simulink model "controller_v13"  (R2020b)
settings: Solver=ode4  StartTime=0.0  StopTime=inf  RelTol=1e-3
undefined symbols (not defined in the file): ctr, DiscIntNeverNeededParam, flt, IO397, mdl, rbt, rsim, som, ukf_P0_flat, ukf_prediction_time, ukf_s0, ukf_sys, ukf_use_prediction
libraries: simulink x31, slrealtimeloglib x5, slrealtimeseriallib x5, speedgoatlib_fpga_analog_io x4, slrealtimetgmanagement x3, speedgoatlib_fpga x2, speedgoatlib_fpga_dio x1, slrealtimeutilitieslib x1
(part 1 of 5)
settings Model: SimulationMode=external  Creator=SMRL  LastModifiedBy=SMRL
settings SolverCC: ConcurrentTasks=on  PositivePriorityOrder=on  AutoInsertRateTranBlk=on
settings DataIOCC: DSMLogging=off
settings OptimizationCC: BlockReduction=off  OptimizeBlockIOStorage=off
settings DebuggingCC: TasksWithSamePriorityMsg=none
settings HardwareCC: ProdBitPerLong=64  ProdLongLongMode=on  ProdHWDeviceType=Intel->x86-64 (Linux 64)
settings RTWCC: Description=Simulink Real-Time  SystemTargetFile=slrealtime.tlc  TemplateMakefile=slrealtime_default_tmf  Toolchain=Simulink Real-Time Toolchain  BuildConfiguration=Faster Runs  CodeExecutionProfiling=on  TargetLang=C++

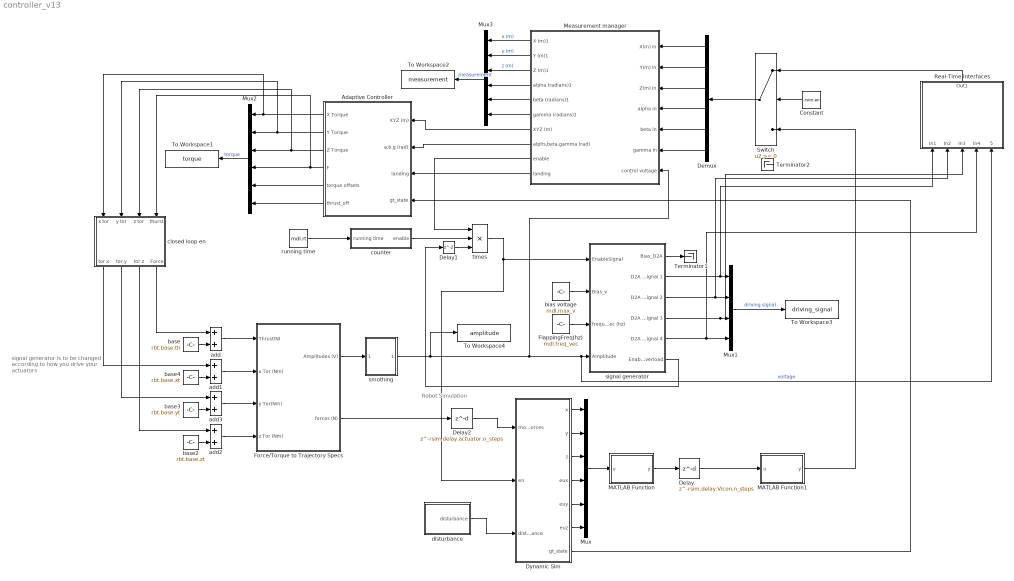
== system controller_v13 ==
  note: Robot Simulation
  note: signal generator is to be changed
      | according to how you drive your
      | actuators
  Adaptive Controller : Subsystem
  Constant : Constant  Value=-rsim.en
  Delay : Delay  DelayLength=rsim.delay.Vicon.n_steps  InitialCondition=rsim.delay.Vicon.init_val
  Delay1 : Delay  InitialCondition=1
  Delay2 : Delay  DelayLength=rsim.delay.actuator.n_steps  InitialCondition=rsim.delay.actuator.init_val
  Demux : Demux  Outputs=6
  Dynamic Sim : Subsystem  TreatAsAtomicUnit=on  SystemSampleTime=rsim.mdl.T
  FlappingFreq(hz) : Constant  Value=mdl.freq_vec  SampleTime=-1
  Force/Torque to Trajectory Specs : Subsystem
  MATLAB Function : MATLAB Function  TreatAsAtomicUnit=on  SystemSampleTime=0.001
  MATLAB Function1 : MATLAB Function  TreatAsAtomicUnit=on  SystemSampleTime=1/1000
  Measurement manager : Subsystem
  Mux : Mux  Inputs=6
  Mux1 : Mux
  Mux2 : Mux  Inputs=6
  Mux3 : Mux  Inputs=6
  Real-Time Interfaces : Subsystem
  Switch : Switch
  Terminator1 : Terminator
  Terminator2 : Terminator
  To Workspace1 : ToWorkspace  VariableName=torque  SaveFormat=Timeseries  SampleTime=-1
  To Workspace2 : ToWorkspace  VariableName=measurement  SaveFormat=Timeseries  SampleTime=-1
  To Workspace3 : ToWorkspace  VariableName=driving_signal  SaveFormat=Timeseries  SampleTime=-1
  To Workspace4 : ToWorkspace  VariableName=amplitude  SaveFormat=Timeseries  SampleTime=-1
  add{,1..3} (4 alike) : Sum
  base : Constant  Value=rbt.base.th
  base2 : Constant  Value=rbt.base.zt
  base3 : Constant  Value=rbt.base.yt
  base4 : Constant  Value=rbt.base.xt
  bias voltage : Constant  Value=mdl.max_v
  closed loop en : Subsystem
  counter : Subsystem
  disturbance : Subsystem  TreatAsAtomicUnit=on  SystemSampleTime=rsim.mdl.T
  running time : Constant  Value=mdl.rt  SampleTime=-1
  signal generator : Subsystem  TreatAsAtomicUnit=on  SystemSampleTime=mdl.T_high
  smothing : Subsystem
  times : Product  Inputs=3  RndMeth=Zero
  wires:
  add3/1 -> Force/Torque to Trajectory Specs/3(y Tor(Nm))
  Force/Torque to Trajectory Specs/2(forces (N)) -> Delay2/1
  Adaptive Controller/3(Z Torque) -> closed loop en/3(z tor), Mux2/3
  Mux3/1 -> To Workspace2/1  "measurement"
  Adaptive Controller/2(Y Torque) -> closed loop en/2(y tor), Mux2/2
  Adaptive Controller/1(X Torque) -> closed loop en/1(x tor), Mux2/1
  signal generator/5(D2A DriveSignal 4) -> Mux1/4, Real-Time Interfaces/4(In4)
  Adaptive Controller/5(" torque offsets") -> Mux2/5
  Measurement manager/5(beta (radians)1) -> Mux3/5
  signal generator/4(D2A DriveSignal 3) -> Real-Time Interfaces/3(In3), Mux1/3
  Adaptive Controller/4(" F") -> closed loop en/4(thurst), Mux2/4
  Measurement manager/6(gamma (radians)1) -> Mux3/6
  add2/1 -> Force/Torque to Trajectory Specs/4(z Tor (Nm))
  Measurement manager/4(alpha (radians)1) -> Mux3/4
  Adaptive Controller/6(thrust_off) -> Mux2/6
  closed loop en/1(tor x) -> add1/1
  base3/1 -> add3/2
  base2/1 -> add2/2
  Mux1/1 -> To Workspace3/1  "driving signal"
  closed loop en/4(Force) -> add/1
  base/1 -> add/2
  Measurement manager/8(alphs,beta,gamma (rad)) -> Adaptive Controller/2(a,b,g (rad))
  signal generator/2(D2A DriveSignal 1) -> Real-Time Interfaces/1(In1), Mux1/1
  closed loop en/2(tor y) -> add3/1
  signal generator/3(D2A DriveSignal 2) -> Mux1/2, Real-Time Interfaces/2(In2)
  Force/Torque to Trajectory Specs/1(Amplitudes (V)) -> smothing/1(amp)
  FlappingFreq(hz)/1 -> signal generator/3(frequency_vec (hz))
  Measurement manager/1(X (m)1) -> Mux3/1  "x (m)"
  Measurement manager/7(XYZ (m)) -> Adaptive Controller/1(XYZ (m))
  Measurement manager/3(Z (m)1) -> Mux3/3  "z (m)"
  base4/1 -> add1/2
  closed loop en/3(tor z) -> add2/1
  add1/1 -> Force/Torque to Trajectory Specs/2(x Tor (Nm))
  bias voltage/1 -> signal generator/2(Bias_v)
  counter/1(enable) -> times/2
  add/1 -> Force/Torque to Trajectory Specs/1(Thrust(N))
  Measurement manager/2(Y (m)1) -> Mux3/2  "y (m)"
  running time/1 -> counter/1(running time)
  Mux2/1 -> To Workspace1/1  "torque"
  signal generator/1(Bias_D2A) -> Terminator1/1
  Dynamic Sim/3(z) -> Mux/3
  Dynamic Sim/2(y) -> Mux/2
  Dynamic Sim/1(x) -> Mux/1
  Dynamic Sim/4(eux) -> Mux/4
  Dynamic Sim/5(euy) -> Mux/5
  Dynamic Sim/6(euz) -> Mux/6
  Demux/1 -> Measurement manager/1(X(m) in)
  Demux/2 -> Measurement manager/2(Y(m) in)
  Demux/3 -> Measurement manager/3(Z(m) in)
  Demux/4 -> Measurement manager/4(alpha in)
  Demux/5 -> Measurement manager/5(beta in)
  Demux/6 -> Measurement manager/6(gamma in)
  Constant/1 -> Switch/2
  disturbance/1(disturbance) -> Dynamic Sim/3(disturbance)
  Switch/1 -> Demux/1
  Delay/1 -> MATLAB Function1/1(u)
  Measurement manager/10(landing) -> Adaptive Controller/3(landing)
  signal generator/6(Enable overload) -> Delay1/1
  Delay1/1 -> times/3
  smothing/1(control voltage) -> Real-Time Interfaces/5(voltage), signal generator/4(Amplitude), Measurement manager/7(control voltage), To Workspace4/1  "voltage"
  Measurement manager/9(enable) -> times/1
  Mux/1 -> MATLAB Function/1(u)
  MATLAB Function/1(y) -> Delay/1
  MATLAB Function1/1(y) -> Switch/3
  Delay2/1 -> Dynamic Sim/1(module forces)
  Dynamic Sim/7(gt_state) -> Adaptive Controller/4(gt_state)
  times/1 -> Dynamic Sim/2(en), signal generator/1(EnableSignal)
  Real-Time Interfaces/1(Out1) -> Switch/1

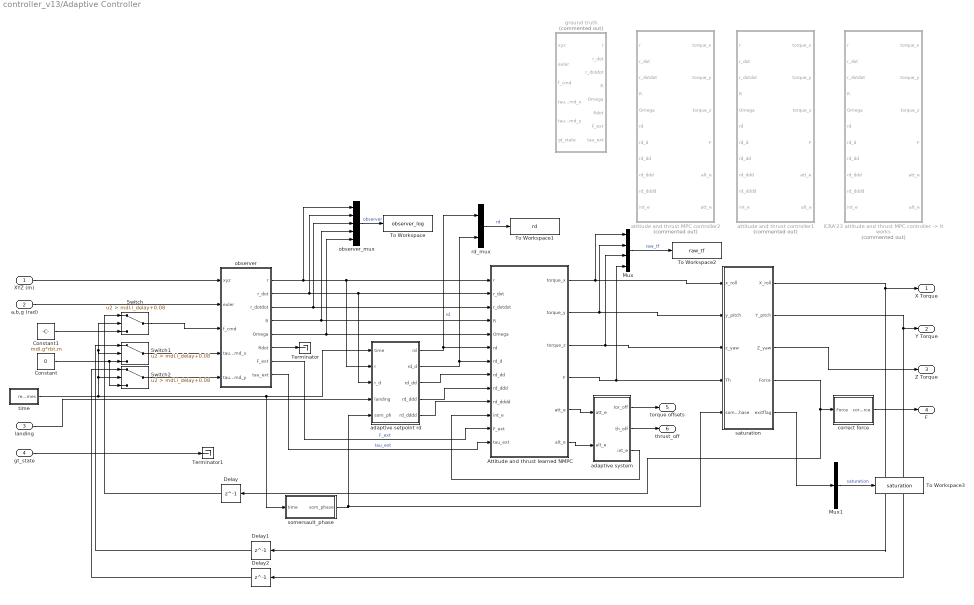
== system controller_v13/Adaptive Controller ==
  XYZ (m) : Inport
  a,b,g (rad) : Inport  Port=2
  landing : Inport  Port=3
  gt_state : Inport  Port=4
  Attitude and thrust learned NMPC : Subsystem
  Constant : Constant  Value=0
  Constant1 : Constant  Value=mdl.g*rbt.m
  Delay : Delay  DelayLength=1
  Delay1 : Delay  DelayLength=1
  Delay2 : Delay  DelayLength=1
  "ICRA'23 attitude and thrust MPC controller -> It works" : Subsystem  Commented=on
  Mux : Mux
  Mux1 : Mux  Inputs=1
  Switch : Switch  Criteria=u2 > Threshold  Threshold=mdl.i_delay+0.08
  Switch1 : Switch  Criteria=u2 > Threshold  Threshold=mdl.i_delay+0.08
  Switch2 : Switch  Criteria=u2 > Threshold  Threshold=mdl.i_delay+0.08
  Terminator : Terminator
  Terminator1 : Terminator
  To Workspace : ToWorkspace  VariableName=observer_log  SaveFormat=Timeseries  SampleTime=-1
  To Workspace1 : ToWorkspace  VariableName=rd  SaveFormat=Timeseries  SampleTime=-1
  To Workspace2 : ToWorkspace  VariableName=raw_tf  SaveFormat=Timeseries  SampleTime=-1
  To Workspace3 : ToWorkspace  VariableName=saturation  SaveFormat=Timeseries  SampleTime=-1
  adaptive setpoint rd : MATLAB Function  TreatAsAtomicUnit=on  SystemSampleTime=mdl.T
  adaptive system : Subsystem
  attitude and thrust MPC controller2 : Subsystem  Commented=on
  attitude and thrust controller1 : Subsystem  Commented=on
  correct force : MATLAB Function  TreatAsAtomicUnit=on
  ground truth : Subsystem  Commented=on
  observer : Subsystem
  observer_mux : Mux  Inputs=5
  rd_mux : Mux  Inputs=2
  saturation : MATLAB Function  TreatAsAtomicUnit=on  SystemSampleTime=mdl.T
  somersault_phase : MATLAB Function  TreatAsAtomicUnit=on
  time : Subsystem
  X Torque : Outport
  Y Torque : Outport  Port=2
  Z Torque : Outport  Port=3
  " F" : Outport  Port=4
  " torque offsets" : Outport  Port=5
  thrust_off : Outport  Port=6
  wires:
  XYZ (m)/1 -> observer/1(xyz)
  observer/2(r_dot) -> Attitude and thrust learned NMPC/2(r_dot), adaptive setpoint rd/3(r_d), observer_mux/2
  observer/3(r_dotdot) -> Attitude and thrust learned NMPC/3(r_dotdot), observer_mux/3
  a,b,g (rad)/1 -> observer/2(euler)
  observer/4(R) -> Attitude and thrust learned NMPC/4(R), observer_mux/4
  saturation/1(X_roll) -> Delay1/1, X Torque/1
  saturation/2(Y_pitch) -> Delay2/1, Y Torque/1
  saturation/3(Z_yaw) -> Z Torque/1
  saturation/4(Force) -> Delay/1, correct force/1(Force)
  Attitude and thrust learned NMPC/4(F) -> Mux/4, saturation/4(Th)
  Attitude and thrust learned NMPC/5(att_e) -> adaptive system/1(att_e)
  adaptive system/1(" tor_off") -> " torque offsets"/1
  adaptive system/2(th_off) -> thrust_off/1
  adaptive system/3(int_e) -> Attitude and thrust learned NMPC/11(int_e)
  adaptive setpoint rd/1(rd) -> Attitude and thrust learned NMPC/6(rd), rd_mux/1  "rd"
  adaptive setpoint rd/2(rd_d) -> Attitude and thrust learned NMPC/7(rd_d), rd_mux/2
  adaptive setpoint rd/3(rd_dd) -> Attitude and thrust learned NMPC/8(rd_dd)
  adaptive setpoint rd/4(rd_ddd) -> Attitude and thrust learned NMPC/9(rd_ddd)
  adaptive setpoint rd/5(rd_dddd) -> Attitude and thrust learned NMPC/10(rd_dddd)
  time/1(real times) -> Switch2/2, Switch/2, Switch1/2, somersault_phase/1(time), adaptive setpoint rd/1(time)
  Attitude and thrust learned NMPC/3(torque_z) -> Mux/3, saturation/3(z_yaw)
  Attitude and thrust learned NMPC/2(torque_y) -> Mux/2, saturation/2(y_pitch)
  Attitude and thrust learned NMPC/1(torque_x) -> Mux/1, saturation/1(x_roll)
  observer/6(Rdot) -> Terminator/1
  observer/5(Omega) -> Attitude and thrust learned NMPC/5(Omega), observer_mux/5
  Attitude and thrust learned NMPC/6(alt_e) -> adaptive system/2(alt_e)
  somersault_phase/1(som_phase) -> saturation/5(som_phase), adaptive setpoint rd/5(som_ph)
  landing/1 -> adaptive setpoint rd/4(landing)
  observer_mux/1 -> To Workspace/1  "observer"
  rd_mux/1 -> To Workspace1/1  "rd"
  Delay/1 -> Switch/1
  observer/1(r) -> Attitude and thrust learned NMPC/1(r), adaptive setpoint rd/2(r), observer_mux/1
  Delay1/1 -> Switch1/1
  Delay2/1 -> Switch2/1
  Constant/1 -> Switch2/3, Switch1/3
  Switch1/1 -> observer/4(tau_cmd_x)
  Switch/1 -> observer/3(f_cmd)
  Constant1/1 -> Switch/3
  observer/7(F_ext) -> Attitude and thrust learned NMPC/12(F_ext)  "F_ext"
  observer/8(tau_ext) -> Attitude and thrust learned NMPC/13(tau_ext)  "tau_ext"
  gt_state/1 -> Terminator1/1
  Switch2/1 -> observer/5(tau_cmd_y)
  Mux/1 -> To Workspace2/1  "raw_tf"
  saturation/5(exitflag) -> Mux1/1
  Mux1/1 -> To Workspace3/1  "saturation"
  correct force/1(corrected_force) -> " F"/1

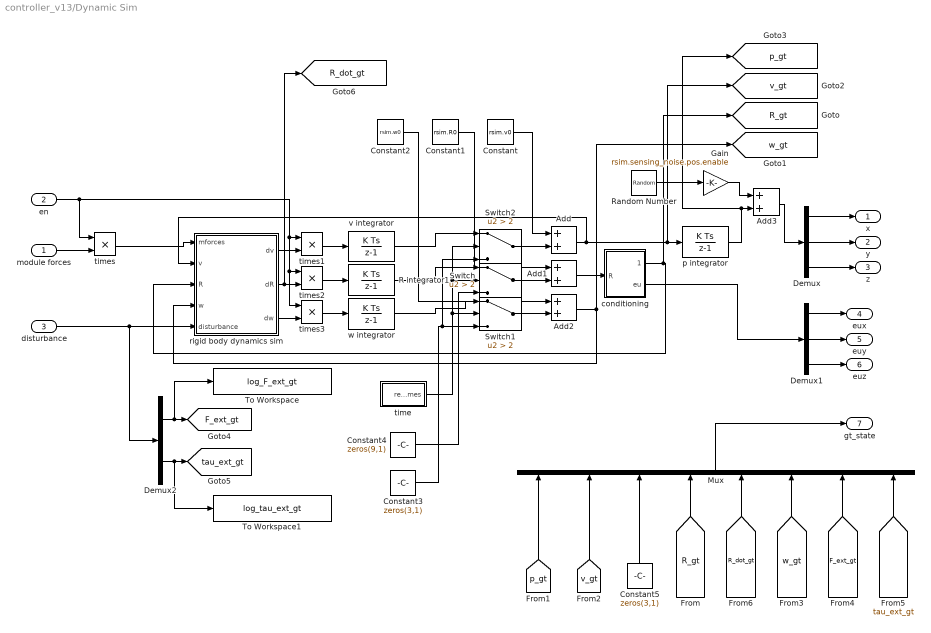
== system controller_v13/Dynamic Sim ==
  module forces : Inport
  en : Inport  Port=2
  disturbance : Inport  Port=3
  Add{,1..3} (4 alike) : Sum
  Constant : Constant  Value=rsim.v0
  Constant1 : Constant  Value=rsim.R0
  Constant2 : Constant  Value=rsim.w0
  Constant3 : Constant  Value=zeros(3,1)
  Constant4 : Constant  Value=zeros(9,1)
  Constant5 : Constant  Value=zeros(3,1)
  Demux : Demux  Outputs=3
  Demux1 : Demux  Outputs=3
  Demux2 : Demux  Outputs=[3, 3]
  Gain : Gain  Gain=rsim.sensing_noise.pos.enable
  Mux : Mux  Inputs=8
  R integrator1 : DiscreteIntegrator  gainval=1  SampleTime=-1  UpperSaturationLimit=1  LowerSaturationLimit=0  ICPrevOutput=DiscIntNeverNeededParam  ICPrevScaledInput=DiscIntNeverNeededParam
  Random Number : RandomNumber  Mean=zeros(3,1)  Variance=rsim.sensing_noise.pos_sigma.^2  SampleTime=rsim.mdl.T
  Switch : Switch  Criteria=u2 > Threshold  Threshold=2
  Switch1 : Switch  Criteria=u2 > Threshold  Threshold=2
  Switch2 : Switch  Criteria=u2 > Threshold  Threshold=2
  To Workspace : ToWorkspace  VariableName=log_F_ext_gt  SaveFormat=Timeseries  SampleTime=-1
  To Workspace1 : ToWorkspace  VariableName=log_tau_ext_gt  SaveFormat=Timeseries  SampleTime=-1
  conditioning : MATLAB Function  TreatAsAtomicUnit=on
  p integrator : DiscreteIntegrator  gainval=1  InitialCondition=rsim.p0  SampleTime=-1  UpperSaturationLimit=1  LowerSaturationLimit=0  ICPrevOutput=DiscIntNeverNeededParam  ICPrevScaledInput=DiscIntNeverNeededParam
  rigid body dynamics sim : MATLAB Function  TreatAsAtomicUnit=on
  time : Subsystem
  times{,1..3} (4 alike) : Product  RndMeth=Zero
  v integrator : DiscreteIntegrator  gainval=1  SampleTime=-1  UpperSaturationLimit=1  LowerSaturationLimit=0  ICPrevOutput=DiscIntNeverNeededParam  ICPrevScaledInput=DiscIntNeverNeededParam
  w integrator : DiscreteIntegrator  gainval=1  SampleTime=-1  UpperSaturationLimit=1  LowerSaturationLimit=0  ICPrevOutput=DiscIntNeverNeededParam  ICPrevScaledInput=DiscIntNeverNeededParam
  x : Outport  VectorParamsAs1DForOutWhenUnconnected=off
  y : Outport  Port=2  VectorParamsAs1DForOutWhenUnconnected=off
  z : Outport  Port=3  VectorParamsAs1DForOutWhenUnconnected=off
  eux : Outport  Port=4  VectorParamsAs1DForOutWhenUnconnected=off
  euy : Outport  Port=5  VectorParamsAs1DForOutWhenUnconnected=off
  euz : Outport  Port=6  VectorParamsAs1DForOutWhenUnconnected=off
  gt_state : Outport  Port=7
  tag scope: F_ext_gt=global, R_dot_gt=global, R_gt=global, p_gt=global, tau_ext_gt=global, v_gt=global, w_gt=global
  wires:
  Demux1/1 -> eux/1
  Demux1/2 -> euy/1
  Demux/3 -> z/1
  conditioning/2(eu) -> Demux1/1
  conditioning/1(R_norm_flat) -> [R_gt], rigid body dynamics sim/3(R)
  p integrator/1 -> [p_gt], Add3/2
  Demux1/3 -> euz/1
  Demux/1 -> x/1
  Demux/2 -> y/1
  Constant/1 -> Add/1
  Constant1/1 -> Add1/1
  Constant2/1 -> Add2/1
  Add1/1 -> conditioning/1(R)
  Add2/1 -> [w_gt], rigid body dynamics sim/4(w)
  Add/1 -> rigid body dynamics sim/2(v), [v_gt], p integrator/1
  en/1 -> times2/1, times3/1, times1/1, times/1
  module forces/1 -> times/2
  times/1 -> rigid body dynamics sim/1(mforces)
  times1/1 -> v integrator/1
  rigid body dynamics sim/1(dv) -> times1/2
  rigid body dynamics sim/2(dR) -> [R_dot_gt], times2/2
  rigid body dynamics sim/3(dw) -> times3/2
  times2/1 -> R integrator1/1
  times3/1 -> w integrator/1
  disturbance/1 -> Demux2/1, rigid body dynamics sim/5(disturbance)
  Random Number/1 -> Gain/1
  Gain/1 -> Add3/1
  Add3/1 -> Demux/1
  Switch2/1 -> Add/2
  Switch/1 -> Add1/2
  Switch1/1 -> Add2/2
  time/1(real times) -> Switch1/2, Switch2/2, Switch/2
  v integrator/1 -> Switch2/1
  R integrator1/1 -> Switch/1
  w integrator/1 -> Switch1/1
  Constant4/1 -> Switch/3
  Constant3/1 -> Switch2/3, Switch1/3
  Demux2/1 -> To Workspace/1, [F_ext_gt]
  Demux2/2 -> To Workspace1/1, [tau_ext_gt]
  [p_gt] -> Mux/1
  [v_gt] -> Mux/2
  Constant5/1 -> Mux/3
  [R_gt] -> Mux/4
  [R_dot_gt] -> Mux/5
  [w_gt] -> Mux/6
  [F_ext_gt] -> Mux/7
  [tau_ext_gt] -> Mux/8
  Mux/1 -> gt_state/1

== system controller_v13/Force//Torque to Trajectory Specs ==
  Thrust(N) : Inport
  x Tor (Nm) : Inport  Port=2
  y Tor(Nm) : Inport  Port=3
  z Tor (Nm) : Inport  Port=4
  force/torque to module thrust : Subsystem
  nominal desired voltage : Subsystem
  Amplitudes (V) : Outport
  forces (N) : Outport  Port=2
  wires:
  Thrust(N)/1 -> force/torque to module thrust/1(thrust)
  y Tor(Nm)/1 -> force/torque to module thrust/3(y Tq)
  z Tor (Nm)/1 -> force/torque to module thrust/4(z Tq)
  force/torque to module thrust/1(module thrusts (1-4)) -> forces (N)/1, nominal desired voltage/1(Force)
  x Tor (Nm)/1 -> force/torque to module thrust/2(x Tq)
  nominal desired voltage/1(Voltages) -> Amplitudes (V)/1

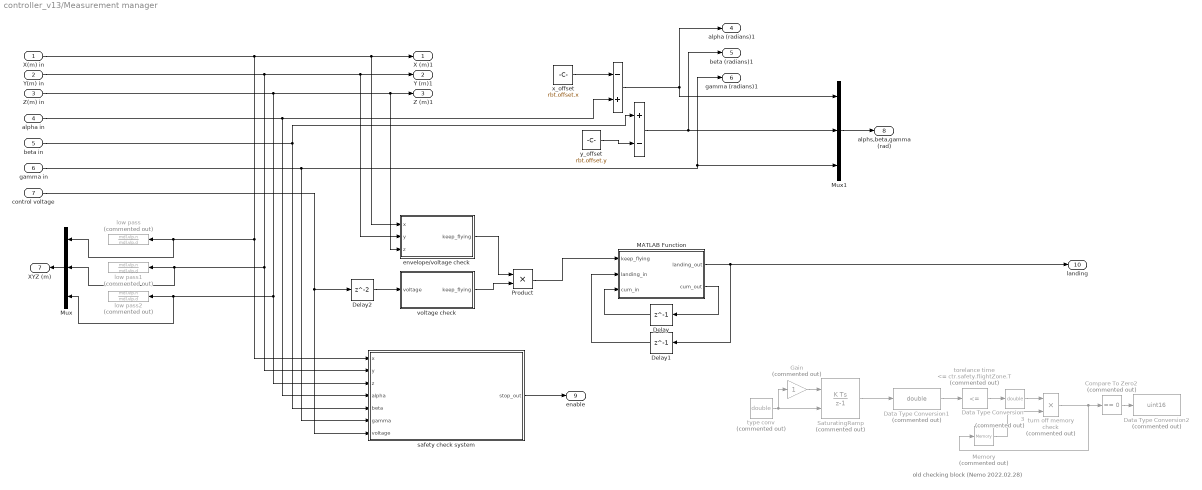
== system controller_v13/Measurement manager ==
  note: old checking block (Nemo 2022.02.28)
  X(m) in : Inport
  Y(m) in : Inport  Port=2
  Z(m) in : Inport  Port=3
  alpha in : Inport  Port=4
  beta in : Inport  Port=5
  gamma in : Inport  Port=6
  control voltage : Inport  Port=7
  " " : Sum  Inputs=-+
  "  " : Sum  Inputs=+-
  Compare To Zero2 : simulink/Logic and Bit Operations/Compare To Zero  Commented=on  relop===  OutDataTypeStr=uint8
  Data Type Conversion1 : DataTypeConversion  Commented=on  OutDataTypeStr=double
  Data Type Conversion2 : DataTypeConversion  Commented=on  OutDataTypeStr=uint16
  Data Type Conversion3 : DataTypeConversion  Commented=on  OutDataTypeStr=double
  Delay : Delay  DelayLength=1
  Delay1 : Delay  DelayLength=1
  Delay2 : Delay
  Gain : Gain  Commented=on
  MATLAB Function : MATLAB Function  TreatAsAtomicUnit=on
  Memory : Memory  Commented=on  InitialCondition=1
  Mux : Mux  Inputs=3
  Mux1 : Mux  Inputs=3
  Product : Product
  SaturatingRamp : DiscreteIntegrator  Commented=on  gainval=1  ExternalReset=falling  SampleTime=-1  UpperSaturationLimit=1  LowerSaturationLimit=0  ICPrevOutput=DiscIntNeverNeededParam  ICPrevScaledInput=DiscIntNeverNeededParam
  envelope/voltage check : MATLAB Function  TreatAsAtomicUnit=on
  low pass : DiscreteTransferFcn  Commented=on  Numerator=mdl.vlp.n  Denominator=mdl.vlp.d
  low pass1 : DiscreteTransferFcn  Commented=on  Numerator=mdl.vlp.n  Denominator=mdl.vlp.d
  low pass2 : DiscreteTransferFcn  Commented=on  Numerator=mdl.vlp.n  Denominator=mdl.vlp.d
  safety check system : Subsystem
  torelance time : simulink/Logic and Bit Operations/Compare To Constant  Commented=on  relop=<=  const=ctr.safety.flightZone.T  OutDataTypeStr=uint8
  turn off memory check : Product  Commented=on  RndMeth=Zero
  type conv : DataTypeConversion  Commented=on  OutDataTypeStr=double
  voltage check : MATLAB Function  TreatAsAtomicUnit=on  SystemSampleTime=mdl.T
  x_offset : Constant  Value=rbt.offset.x
  y_offset : Constant  Value=rbt.offset.y
  X (m)1 : Outport
  Y (m)1 : Outport  Port=2
  Z (m)1 : Outport  Port=3
  alpha (radians)1 : Outport  Port=4
  beta (radians)1 : Outport  Port=5
  gamma (radians)1 : Outport  Port=6
  XYZ (m) : Outport  Port=7
  alphs,beta,gamma (rad) : Outport  Port=8
  enable : Outport  Port=9
  landing : Outport  Port=10
  wires:
  X(m) in/1 -> safety check system/1(x), Mux/1, low pass/1, envelope/voltage check/1(x), X (m)1/1
  Y(m) in/1 -> safety check system/2(y), Mux/2, low pass1/1, envelope/voltage check/2(y), Y (m)1/1
  Z(m) in/1 -> safety check system/3(z), Mux/3, low pass2/1, envelope/voltage check/3(z), Z (m)1/1
  alpha in/1 -> safety check system/4(alpha), " "/2
  beta in/1 -> "  "/1, safety check system/5(beta)
  Mux/1 -> XYZ (m)/1
  Mux1/1 -> alphs,beta,gamma (rad)/1
  y_offset/1 -> "  "/2
  x_offset/1 -> " "/1
  control voltage/1 -> Delay2/1, safety check system/7(voltage)
  safety check system/1(stop_out) -> enable/1
  Gain/1 -> SaturatingRamp/1
  Data Type Conversion3/1 -> turn off memory check/1
  Data Type Conversion1/1 -> torelance time/1
  type conv/1 -> SaturatingRamp/2, Gain/1
  SaturatingRamp/1 -> Data Type Conversion1/1
  torelance time/1 -> Data Type Conversion3/1
  turn off memory check/1 -> Compare To Zero2/1, Memory/1
  Memory/1 -> turn off memory check/2
  Compare To Zero2/1 -> Data Type Conversion2/1
  " "/1 -> Mux1/1, alpha (radians)1/1
  "  "/1 -> beta (radians)1/1, Mux1/2
  gamma in/1 -> Mux1/3, gamma (radians)1/1, safety check system/6(gamma)
  Delay/1 -> MATLAB Function/3(cum_in)
  MATLAB Function/2(cum_out) -> Delay/1
  MATLAB Function/1(landing_out) -> Delay1/1, landing/1
  Delay1/1 -> MATLAB Function/2(landing_in)
  envelope/voltage check/1(keep_flying) -> Product/1
  Delay2/1 -> voltage check/1(voltage)
  voltage check/1(keep_flying) -> Product/2
  Product/1 -> MATLAB Function/1(keep_flying)

== system controller_v13/Real-Time Interfaces ==
  In1 : Inport
  In2 : Inport  Port=2
  In3 : Inport  Port=3
  In4 : Inport  Port=4
  voltage : Inport  Port=5
  Cast To Double : DataTypeConversion  OutDataTypeStr=double
  Constant1 : Constant  Value=mdl.i_delay
  Digital output : speedgoatlib_fpga_dio/Digital output  id=2  chan=[7]  init=[0]  reset=[0]  vectorizeInput=off  ts=mdl.T  pciSlot=[11,0]  board=IO397-50k
      settings: SourceProductName=Simulink Real-Time: Speedgoat I/O Driver Library
  IO397 Analog Output : speedgoatlib_fpga_analog_io/IO397 Analog Output  id=1  chan=1:2  initVal=0  resetVal=0  ts=-1  pciSlot=[6,0]  board=IO397-50k  span=+10.8 V
      settings: SourceProductName=Simulink Real-Time: Speedgoat Library
  IO397 Analog Output1 : speedgoatlib_fpga_analog_io/IO397 Analog Output  id=2  chan=1:2  initVal=0  resetVal=0  ts=-1  pciSlot=[11,0]  board=IO397-50k  span=+10.8 V
      settings: SourceProductName=Simulink Real-Time: Speedgoat Library
  Mux4 : Mux  Inputs=6
  Overload Options : slrealtimetgmanagement/Overload Options  startupDur=600  startupDurSrc=Tunable Parameter  maxOverload=10  maxOverloadSrc=Tunable Parameter  TETFlag=on
      settings: SourceProductBaseCode=XP
  Relational Operator : RelationalOperator  Operator=>  OutDataTypeStr=boolean  RndMeth=Simplest
  Setup : speedgoatlib_fpga/Setup/Setup  board=IO397-50k  id=2  device_id=2  frontIO=None  rearIO=None  bitstreamFile=speedgoat_IO397_50k_all_io_2.mat  rev=2.1  timestamp_string=06/12/19 11:07:30  fpgaFreq=75 MHz  fpgaTick=13.33 ns  ProgSpiFlash=off  ProgBPIFlash=off  pciSlot=[11,0]  PullRPort0=pull-up 3.3V  VioPort0=3.3V  PullRPort1=pull-up 3.3V  VioPort1=3.3V  PullRPort2=pull-up 3.3V  VioPort2=3.3V  PullRPort3=pull-up 3.3V  VioPort3=3.3V  PullRPort4=pull-up 3.3V  VioPort4=3.3V  PullRPort5=pull-up 3.3V  VioPort5=3.3V  PullRPort6=pull-up 3.3V  VioPort6=3.3V  PullRPort15=pull-up 3.3V  PullRPort31=pull-up 3.3V  PullRPort47=pull-up 3.3V  PullRPort63=pull-up 3.3V
      settings: SourceProductName=Simulink Real-Time: Speedgoat Library
  Setup1 : speedgoatlib_fpga/Setup/Setup  board=IO397-50k  id=1  device_id=1  frontIO=None  rearIO=None  bitstreamFile=speedgoat_IO397_50k_all_io_2.mat  rev=2.1  timestamp_string=06/12/19 11:07:30  fpgaFreq=75 MHz  fpgaTick=13.33 ns  ProgSpiFlash=off  ProgBPIFlash=off  pciSlot=[6,0]  PullRPort0=pull-up 3.3V  VioPort0=3.3V  PullRPort1=pull-up 3.3V  VioPort1=3.3V  PullRPort2=pull-up 3.3V  VioPort2=3.3V  PullRPort3=pull-up 3.3V  VioPort3=3.3V  PullRPort4=pull-up 3.3V  VioPort4=3.3V  PullRPort5=pull-up 3.3V  VioPort5=3.3V  PullRPort6=pull-up 3.3V  VioPort6=3.3V  PullRPort15=pull-up 3.3V  PullRPort31=pull-up 3.3V  PullRPort47=pull-up 3.3V  PullRPort63=pull-up 3.3V
      settings: SourceProductName=Simulink Real-Time: Speedgoat Library
  Terminator : Terminator
  Terminator3 : Terminator
  Vicon Measurements : Subsystem
  constant : Constant
  time : DiscreteIntegrator  gainval=1  SampleTime=-1  UpperSaturationLimit=1  LowerSaturationLimit=0  ICPrevOutput=DiscIntNeverNeededParam  ICPrevScaledInput=DiscIntNeverNeededParam
  z Amplifier Measurement : Subsystem
  Out1 : Outport
  wires:
  In1/1 -> IO397 Analog Output/1
  voltage/1 -> Overload Options/1
  Vicon Measurements/4(alpha (radians)) -> Mux4/4
  Mux4/1 -> Out1/1
  In4/1 -> IO397 Analog Output1/2
  Vicon Measurements/3(Z (m)) -> Mux4/3
  In2/1 -> IO397 Analog Output/2
  Vicon Measurements/1(X (m)) -> Mux4/1
  constant/1 -> time/1
  Constant1/1 -> Relational Operator/2
  Vicon Measurements/5(beta (radians)) -> Mux4/5
  Vicon Measurements/6(gamma (radians)) -> Mux4/6
  Cast To Double/1 -> Digital output/1
  time/1 -> Relational Operator/1
  Overload Options/2 -> Terminator3/1  "TET"
  In3/1 -> IO397 Analog Output1/1
  Relational Operator/1 -> Cast To Double/1
  Overload Options/1 -> Terminator/1
  Vicon Measurements/2(Y (m)) -> Mux4/2

== system controller_v13/closed loop en ==
  x tor : Inport
  y tor : Inport  Port=2
  z tor : Inport  Port=3
  thurst : Inport  Port=4
  enable : Constant  Value=ctr.en
  enable{1..4} (4 alike) : Product  Inputs=**
  safety1 : Subsystem
  safety2 : Subsystem
  safety3 : Subsystem
  safety4 : Subsystem
  tor x : Outport
  tor y : Outport  Port=2
  tor z : Outport  Port=3
  Force : Outport  Port=4
  wires:
  enable/1 -> enable2/1, enable3/1, enable4/1, enable1/1
  z tor/1 -> enable3/2
  y tor/1 -> enable2/2
  x tor/1 -> enable1/2
  thurst/1 -> enable4/2
  enable1/1 -> safety1/1(In1)
  enable2/1 -> safety2/1(In1)
  enable3/1 -> safety3/1(In1)
  enable4/1 -> safety4/1(In1)
  safety1/1(Out1) -> tor x/1
  safety2/1(Out1) -> tor y/1
  safety3/1(Out1) -> tor z/1
  safety4/1(Out1) -> Force/1

== system controller_v13/counter ==
  running time : Inport
  Add : Sum  Inputs=+-
  Add1 : Sum
  Compare To Zero : simulink/Logic and Bit Operations/Compare To Zero  relop=<  OutDataTypeStr=uint8  ZeroCross=off
  Product2 : Product  RndMeth=Zero
  Relational Operator : RelationalOperator  Operator=>  OutDataTypeStr=boolean  RndMeth=Simplest
  SaturatingRamp : DiscreteIntegrator  gainval=1  SampleTime=-1  UpperSaturationLimit=1  LowerSaturationLimit=0  ICPrevOutput=DiscIntNeverNeededParam  ICPrevScaledInput=DiscIntNeverNeededParam
  Stop Simulation : Stop
  constant : Constant
  start delay compare : simulink/Logic and Bit Operations/Compare To Constant  relop=>  const=mdl.i_delay  OutDataTypeStr=uint8
  enable : Outport
  wires:
  SaturatingRamp/1 -> Relational Operator/1, Add/1, start delay compare/1
  running time/1 -> Add1/2, Add/2
  Add/1 -> Compare To Zero/1
  start delay compare/1 -> Product2/1
  Compare To Zero/1 -> Product2/2
  Product2/1 -> enable/1
  constant/1 -> Add1/1, SaturatingRamp/1
  Relational Operator/1 -> Stop Simulation/1
  Add1/1 -> Relational Operator/2

== system controller_v13/disturbance ==
  note: Force and torque disturbances modeled as a random walk,
      | with an initial mean and some random walk covariance.
      | f_next = f_curr + Normal(mean=0, sd=...)
  Constant : Constant  Value=rsim.dist.pos.en
  Constant1 : Constant  Value=[0;0;0;]
  Constant2 : Constant  Value=rsim.dist.rot.en
  Constant3 : Constant  Value=[0;0;0;]
  Discrete-Time Integrator1 : DiscreteIntegrator  gainval=ones(3,1)  InitialCondition=[rsim.dist.x.mean; rsim.dist.y.mean; rsim.dist.z.mean]  SampleTime=-1  ICPrevOutput=DiscIntNeverNeededParam  ICPrevScaledInput=DiscIntNeverNeededParam
  Discrete-Time Integrator2 : DiscreteIntegrator  gainval=ones(3,1)  InitialCondition=[rsim.dist.wx.mean; rsim.dist.wz.mean; rsim.dist.wz.mean]  SampleTime=-1  ICPrevOutput=DiscIntNeverNeededParam  ICPrevScaledInput=DiscIntNeverNeededParam
  Mux1 : Mux  Inputs=3
  Mux2 : Mux  Inputs=3
  Mux3 : Mux  Inputs=2
  Random Number : RandomNumber  Variance=rsim.dist.x.var  Seed=rsim.dist.x.seed
  Random Number1 : RandomNumber  Variance=rsim.dist.y.var  Seed=rsim.dist.y.seed
  Random Number2 : RandomNumber  Variance=rsim.dist.z.var  Seed=rsim.dist.z.seed
  Random Number3 : RandomNumber  Variance=rsim.dist.wx.var  Seed=rsim.dist.wx.seed
  Random Number4 : RandomNumber  Variance=rsim.dist.wy.var  Seed=rsim.dist.wy.seed
  Random Number5 : RandomNumber  Variance=rsim.dist.wz.var  Seed=rsim.dist.wz.seed
  Switch : Switch  Threshold=1
  Switch1 : Switch  Threshold=1
  disturbance : Outport  VectorParamsAs1DForOutWhenUnconnected=off
  wires:
  Random Number2/1 -> Mux1/3
  Mux1/1 -> Discrete-Time Integrator1/1
  Random Number1/1 -> Mux1/2
  Switch/1 -> Mux3/1
  Constant/1 -> Switch/2
  Constant1/1 -> Switch/3
  Mux2/1 -> Discrete-Time Integrator2/1
  Random Number5/1 -> Mux2/3
  Constant3/1 -> Switch1/3
  Constant2/1 -> Switch1/2
  Random Number4/1 -> Mux2/2
  Random Number3/1 -> Mux2/1
  Switch1/1 -> Mux3/2
  Mux3/1 -> disturbance/1
  Random Number/1 -> Mux1/1
  Discrete-Time Integrator1/1 -> Switch/1
  Discrete-Time Integrator2/1 -> Switch1/1

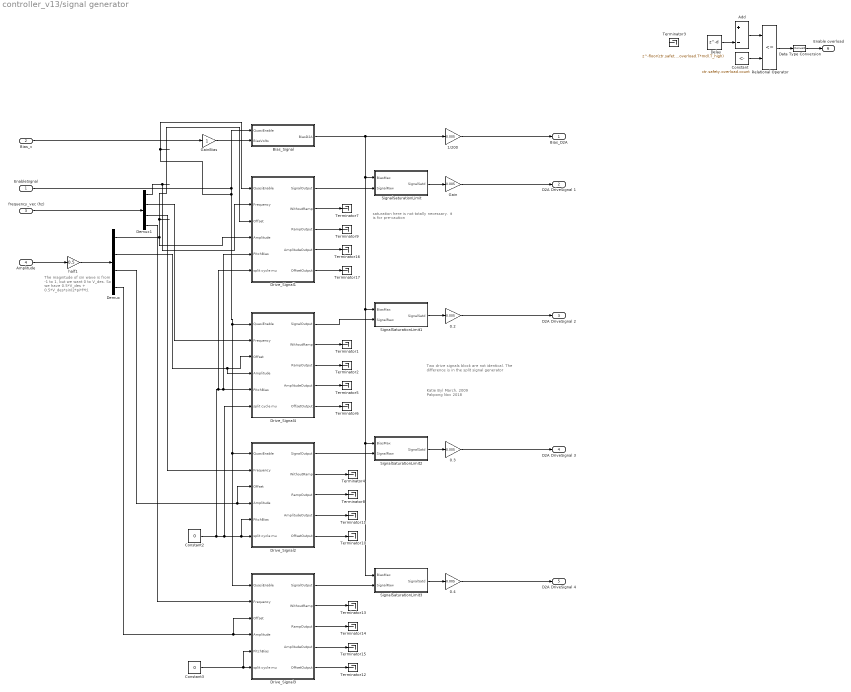
== system controller_v13/signal generator ==
  note: The magnitude of sin wave is from -1 to 1, but we want 0 to V_des. So we have 0.5*V_des + 0.5*V_des*sin(2*pi*f*t).
  note: Katie Byl
      | March, 2009
      |
      | Pakpong
      | Nov 2018
  note: Two drive signals block are not identical.
      | The difference is in the split signal generator
  note: saturation here is not totally necessary.
      | it is for pre-caution
  EnableSignal : Inport
  Bias_v : Inport  Port=2
  frequency_vec (hz) : Inport  Port=3
  Amplitude : Inport  Port=4
  0.2 : Gain  Gain=0.005
  0.3 : Gain  Gain=0.005
  0.4 : Gain  Gain=0.005
  1/200 : Gain  Gain=0.005
  Add : Sum  Inputs=+-
  Bias_Signal : Subsystem
  Constant : Constant  Value=ctr.safety.overload.count
  Constant2 : Constant  Value=0
  Constant3 : Constant  Value=0
  Data Type Conversion : DataTypeConversion
  Delay : Delay  DelayLength=floor(ctr.safety.overload.T*mdl.T_high)  InitialCondition=0
  Demux : Demux
  Demux1 : Demux
  Drive_Signal1 : Subsystem
  Drive_Signal2 : Subsystem
  Drive_Signal3 : Subsystem
  Drive_Signal4 : Subsystem
  Gain : Gain  Gain=0.005
  GainBias : Gain
  Relational Operator : RelationalOperator  Operator=<=  OutDataTypeStr=boolean  RndMeth=Simplest
  SignalSaturationLimit : Subsystem
  SignalSaturationLimit1 : Subsystem
  SignalSaturationLimit2 : Subsystem
  SignalSaturationLimit3 : Subsystem
  Terminator{1..17} (17 alike) : Terminator
  half1 : Gain  Gain=0.5
  Bias_D2A : Outport
  D2A DriveSignal 1 : Outport  Port=2
  D2A DriveSignal 2 : Outport  Port=3
  D2A DriveSignal 3 : Outport  Port=4
  D2A DriveSignal 4 : Outport  Port=5
  Enable overload : Outport  Port=6
  wires:
  Bias_Signal/1(BiasD2A) -> SignalSaturationLimit3/1(BiasMax), SignalSaturationLimit2/1(BiasMax), SignalSaturationLimit1/1(BiasMax), SignalSaturationLimit/1(BiasMax), 1/200/1
  Bias_v/1 -> GainBias/1
  EnableSignal/1 -> Drive_Signal1/1(QuasiEnable), Drive_Signal3/1(QuasiEnable), Drive_Signal2/1(QuasiEnable), Drive_Signal4/1(QuasiEnable), Bias_Signal/1(QuasiEnable)
  SignalSaturationLimit/1(SignalSatd) -> Gain/1
  GainBias/1 -> Bias_Signal/2(BiasVolts)
  SignalSaturationLimit1/1(SignalSatd) -> 0.2/1
  Amplitude/1 -> half1/1
  1/200/1 -> Bias_D2A/1
  Gain/1 -> D2A DriveSignal 1/1
  Drive_Signal3/4(AmplitudeOutput) -> Terminator15/1
  Drive_Signal3/2(WithoutRamp) -> Terminator13/1
  Drive_Signal3/3(RampOutput) -> Terminator14/1
  Drive_Signal3/5(OffsetOutput) -> Terminator12/1
  Drive_Signal2/3(RampOutput) -> Terminator8/1
  Drive_Signal2/4(AmplitudeOutput) -> Terminator11/1
  Drive_Signal3/1(SignalOutput) -> SignalSaturationLimit3/2(SignalRaw)
  Drive_Signal2/5(OffsetOutput) -> Terminator10/1
  Drive_Signal2/2(WithoutRamp) -> Terminator4/1
  Demux/2 -> Drive_Signal4/4(Amplitude), Drive_Signal4/3(Offset)
  Demux/3 -> Drive_Signal2/4(Amplitude), Drive_Signal2/3(Offset)
  Demux/4 -> Drive_Signal3/4(Amplitude), Drive_Signal3/3(Offset)
  Constant2/1 -> Drive_Signal1/6(split cycle mu), Drive_Signal1/5(PitchBias), Drive_Signal4/5(PitchBias), Drive_Signal4/6(split cycle mu), Drive_Signal2/5(PitchBias), Drive_Signal2/6(split cycle mu)
  Constant3/1 -> Drive_Signal3/5(PitchBias), Drive_Signal3/6(split cycle mu)
  0.3/1 -> D2A DriveSignal 3/1
  SignalSaturationLimit2/1(SignalSatd) -> 0.3/1
  0.4/1 -> D2A DriveSignal 4/1
  SignalSaturationLimit3/1(SignalSatd) -> 0.4/1
  Drive_Signal2/1(SignalOutput) -> SignalSaturationLimit2/2(SignalRaw)
  half1/1 -> Demux/1
  frequency_vec (hz)/1 -> Demux1/1
  Demux1/1 -> Drive_Signal1/2(Frequency)
  Demux1/2 -> Drive_Signal4/2(Frequency)
  Demux1/3 -> Drive_Signal2/2(Frequency)
  Demux1/4 -> Drive_Signal3/2(Frequency)
  0.2/1 -> D2A DriveSignal 2/1
  ? -> Delay/1, Add/1  "DrSig count"
  ? -> Terminator3/1  "DrSig TET"
  Delay/1 -> Add/2
  Add/1 -> Relational Operator/1
  Constant/1 -> Relational Operator/2
  Relational Operator/1 -> Data Type Conversion/1
  Data Type Conversion/1 -> Enable overload/1
  Drive_Signal4/1(SignalOutput) -> SignalSaturationLimit1/2(SignalRaw)
  Drive_Signal4/2(WithoutRamp) -> Terminator1/1
  Drive_Signal4/3(RampOutput) -> Terminator2/1
  Drive_Signal4/4(AmplitudeOutput) -> Terminator5/1
  Drive_Signal4/5(OffsetOutput) -> Terminator6/1
  Drive_Signal1/4(AmplitudeOutput) -> Terminator16/1
  Drive_Signal1/1(SignalOutput) -> SignalSaturationLimit/2(SignalRaw)
  Drive_Signal1/2(WithoutRamp) -> Terminator7/1
  Drive_Signal1/5(OffsetOutput) -> Terminator17/1
  Drive_Signal1/3(RampOutput) -> Terminator9/1
  Demux/1 -> Drive_Signal1/3(Offset), Drive_Signal1/4(Amplitude)

== system controller_v13/smothing ==
  amp : Inport
  Delay : Delay  DelayLength=1
  SaturatingRamp : DiscreteIntegrator  gainval=1  SampleTime=-1  UpperSaturationLimit=1  LowerSaturationLimit=0  ICPrevOutput=DiscIntNeverNeededParam  ICPrevScaledInput=DiscIntNeverNeededParam
  constant : Constant
  smoothing : MATLAB Function  TreatAsAtomicUnit=on
  control voltage : Outport
  wires:
  smoothing/1(out_amp) -> Delay/1, control voltage/1
  amp/1 -> smoothing/2(amp)
  Delay/1 -> smoothing/3(amp2)
  constant/1 -> SaturatingRamp/1
  SaturatingRamp/1 -> smoothing/1(time)

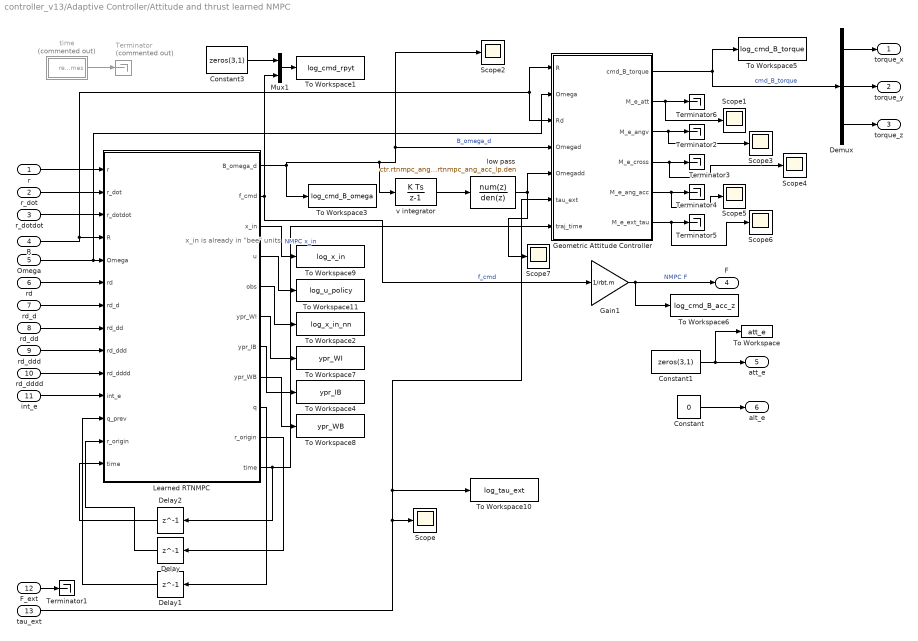
== system controller_v13/Adaptive Controller/Attitude and thrust learned NMPC ==
  note: x_in is already in "bee" units
  r : Inport
  r_dot : Inport  Port=2
  r_dotdot : Inport  Port=3
  R : Inport  Port=4
  Omega : Inport  Port=5  PortDimensions=3
  rd : Inport  Port=6
  rd_d : Inport  Port=7
  rd_dd : Inport  Port=8
  rd_ddd : Inport  Port=9
  rd_dddd : Inport  Port=10
  int_e : Inport  Port=11
  F_ext : Inport  Port=12
  tau_ext : Inport  Port=13
  Constant : Constant  Value=0  VectorParams1D=off
  Constant1 : Constant  Value=zeros(3,1)  VectorParams1D=off
  Constant3 : Constant  Value=zeros(3,1)
  Delay : Delay  DelayLength=1  InitialCondition=zeros(3,1)
  Delay1 : Delay  DelayLength=1  InitialCondition=[0; 0; 0; 1]
  Delay2 : Delay  DelayLength=1  InitialCondition=-mdl.i_delay
  Demux : Demux  Outputs=3
  Gain1 : Gain  Gain=1/rbt.m
  Geometric Attitude Controller : MATLAB Function  TreatAsAtomicUnit=on
  Learned RTNMPC : MATLAB Function  TreatAsAtomicUnit=on
  Mux1 : Mux  Inputs=2
  Scope{,1..7} (8 alike) : Scope
  Terminator : Terminator  Commented=on
  Terminator{1..6} (6 alike) : Terminator
  To Workspace : ToWorkspace  VariableName=att_e  SaveFormat=Timeseries  SampleTime=-1
  To Workspace1 : ToWorkspace  VariableName=log_cmd_rpyt  SaveFormat=Timeseries  SampleTime=-1
  To Workspace10 : ToWorkspace  VariableName=log_tau_ext  SaveFormat=Timeseries  SampleTime=-1
  To Workspace11 : ToWorkspace  VariableName=log_u_policy  SaveFormat=Timeseries  SampleTime=-1
  To Workspace2 : ToWorkspace  VariableName=log_x_in_nn  SaveFormat=Timeseries  SampleTime=-1
  To Workspace3 : ToWorkspace  VariableName=log_cmd_B_omega  SaveFormat=Timeseries  SampleTime=-1
  To Workspace4 : ToWorkspace  VariableName=ypr_IB  SaveFormat=Timeseries  SampleTime=-1
  To Workspace5 : ToWorkspace  VariableName=log_cmd_B_torque  SaveFormat=Timeseries  SampleTime=-1
  To Workspace6 : ToWorkspace  VariableName=log_cmd_B_acc_z  SaveFormat=Timeseries  SampleTime=-1
  To Workspace7 : ToWorkspace  VariableName=ypr_WI  SaveFormat=Timeseries  SampleTime=-1
  To Workspace8 : ToWorkspace  VariableName=ypr_WB  SaveFormat=Timeseries  SampleTime=-1
  To Workspace9 : ToWorkspace  VariableName=log_x_in  SaveFormat=Timeseries  SampleTime=-1
  low pass : DiscreteTransferFcn  Numerator=ctr.rtnmpc_ang_acc_lp.num  Denominator=ctr.rtnmpc_ang_acc_lp.den
  time : Subsystem  Commented=on
  v integrator : DiscreteIntegrator  gainval=1  SampleTime=-1  UpperSaturationLimit=1  LowerSaturationLimit=0  ICPrevOutput=DiscIntNeverNeededParam  ICPrevScaledInput=DiscIntNeverNeededParam
  torque_x : Outport  PortDimensions=1  VectorParamsAs1DForOutWhenUnconnected=off
  torque_y : Outport  Port=2  PortDimensions=1  VectorParamsAs1DForOutWhenUnconnected=off
  torque_z : Outport  Port=3  PortDimensions=1  VectorParamsAs1DForOutWhenUnconnected=off
  F : Outport  Port=4  VectorParamsAs1DForOutWhenUnconnected=off
  att_e : Outport  Port=5  PortDimensions=3  VectorParamsAs1DForOutWhenUnconnected=off
  alt_e : Outport  Port=6  VectorParamsAs1DForOutWhenUnconnected=off
  wires:
  r/1 -> Learned RTNMPC/1(r)
  r_dot/1 -> Learned RTNMPC/2(r_dot)
  r_dotdot/1 -> Learned RTNMPC/3(r_dotdot)
  Omega/1 -> Geometric Attitude Controller/2(Omega), Learned RTNMPC/5(Omega)
  rd/1 -> Learned RTNMPC/6(rd)
  rd_d/1 -> Learned RTNMPC/7(rd_d)
  rd_dd/1 -> Learned RTNMPC/8(rd_dd)
  rd_ddd/1 -> Learned RTNMPC/9(rd_ddd)
  rd_dddd/1 -> Learned RTNMPC/10(rd_dddd)
  int_e/1 -> Learned RTNMPC/11(int_e)
  Constant/1 -> alt_e/1
  Constant1/1 -> att_e/1, To Workspace/1
  Geometric Attitude Controller/1(cmd_B_torque) -> To Workspace5/1, Demux/1  "cmd_B_torque"
  Gain1/1 -> F/1, To Workspace6/1  "NMPC F"
  Mux1/1 -> To Workspace1/1
  Constant3/1 -> Mux1/1
  time/1(real times) -> Terminator/1
  Learned RTNMPC/1(B_omega_d) -> To Workspace3/1, v integrator/1, Scope2/1, Geometric Attitude Controller/4(Omegad)  "B_omega_d"
  Learned RTNMPC/3(x_in) -> To Workspace9/1  "NMPC x_in"
  tau_ext/1 -> Geometric Attitude Controller/6(tau_ext), To Workspace10/1, Scope/1
  Demux/1 -> torque_x/1
  Demux/2 -> torque_y/1
  Demux/3 -> torque_z/1
  Learned RTNMPC/2(f_cmd) -> Gain1/1, Mux1/2  "f_cmd"
  Learned RTNMPC/4(u) -> To Workspace11/1
  Learned RTNMPC/11(time) -> Geometric Attitude Controller/7(traj_time), Delay2/1
  Delay2/1 -> Learned RTNMPC/14("time ")
  Learned RTNMPC/5(obs) -> To Workspace2/1
  Learned RTNMPC/6(ypr_WI) -> To Workspace7/1
  Learned RTNMPC/7(ypr_IB) -> To Workspace4/1
  Learned RTNMPC/8(ypr_WB) -> To Workspace8/1
  F_ext/1 -> Terminator1/1
  Geometric Attitude Controller/3(M_e_angv) -> Scope3/1, Terminator2/1
  Geometric Attitude Controller/4(M_e_cross) -> Scope4/1, Terminator3/1
  Geometric Attitude Controller/5(M_e_ang_acc) -> Scope5/1, Terminator4/1
  Geometric Attitude Controller/6(M_e_ext_tau) -> Scope6/1, Terminator5/1
  Geometric Attitude Controller/2(M_e_att) -> Scope1/1, Terminator6/1
  low pass/1 -> Scope7/1, Geometric Attitude Controller/5(Omegadd)
  v integrator/1 -> low pass/1
  Learned RTNMPC/10(r_origin) -> Delay/1
  Delay/1 -> Learned RTNMPC/13("r_origin ")
  R/1 -> Geometric Attitude Controller/3(Rd), Geometric Attitude Controller/1(R), Learned RTNMPC/4(R)
  Learned RTNMPC/9(q) -> Delay1/1
  Delay1/1 -> Learned RTNMPC/12(q_prev)

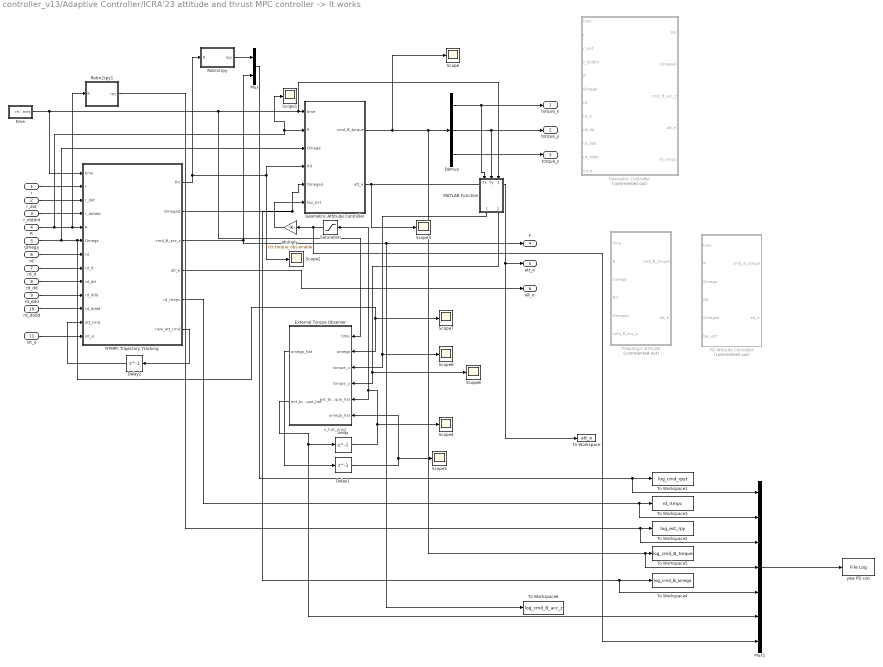
== system controller_v13/Adaptive Controller/ICRA'23 attitude and thrust MPC controller -> It works ==
  note: x_hat_pred
  r : Inport
  r_dot : Inport  Port=2
  r_dotdot : Inport  Port=3
  R : Inport  Port=4
  Omega : Inport  Port=5  PortDimensions=3
  rd : Inport  Port=6
  rd_d : Inport  Port=7
  rd_dd : Inport  Port=8
  rd_ddd : Inport  Port=9
  rd_dddd : Inport  Port=10
  int_e : Inport  Port=11
  Delay : Delay  DelayLength=1  InitialCondition=[ctr.torque_obs.initial_torque.x; ctr.torque_obs.initial_torque.y]  SampleTime=mdl.T
  Delay1 : Delay  DelayLength=1  InitialCondition=[0.0; 0.0]  SampleTime=mdl.T
  Delay2 : Delay  DelayLength=1  InitialCondition=[0.0; 0.0]  SampleTime=mdl.T
  Demux : Demux  Outputs=3
  External Torque Observer : MATLAB Function  TreatAsAtomicUnit=on
  Geometric Attitude Controller : MATLAB Function  TreatAsAtomicUnit=on
  Geometric Controller : MATLAB Function  Commented=on  TreatAsAtomicUnit=on
  MATLAB Function : MATLAB Function  TreatAsAtomicUnit=on
  Multiply : Gain  Gain=ctr.torque_obs.enable
  Mux : Mux  Inputs=2
  Mux1 : Mux  Inputs=7
  PD Atttiude Controller : MATLAB Function  Commented=on  TreatAsAtomicUnit=on
  Pakpong;s atttiude : MATLAB Function  Commented=on  TreatAsAtomicUnit=on
  RTMPC Trajectory Tracking : MATLAB Function  TreatAsAtomicUnit=on
  Rotm2rpy : MATLAB Function  TreatAsAtomicUnit=on
  Rotm2rpy1 : MATLAB Function  TreatAsAtomicUnit=on
  Saturation : Saturate  UpperLimit=1.8*1e-5.*ones(2,1)  LowerLimit=-1.8*1e-5.*ones(2,1)
  Scope{,1..8} (9 alike) : Scope
  To Workspace : ToWorkspace  VariableName=att_e  SaveFormat=Timeseries  SampleTime=-1
  To Workspace1 : ToWorkspace  VariableName=log_cmd_rpyt  SaveFormat=Timeseries  SampleTime=-1
  To Workspace2 : ToWorkspace  VariableName=log_est_rpy  SaveFormat=Timeseries  SampleTime=-1
  To Workspace3 : ToWorkspace  VariableName=rd_rtmpc  SaveFormat=Timeseries  SampleTime=-1
  To Workspace4 : ToWorkspace  VariableName=log_cmd_B_omega  SaveFormat=Timeseries  SampleTime=-1
  To Workspace5 : ToWorkspace  VariableName=log_cmd_B_torque  SaveFormat=Timeseries  SampleTime=-1
  To Workspace6 : ToWorkspace  VariableName=log_cmd_B_acc_z  SaveFormat=Timeseries  SampleTime=-1
  time : Subsystem
  yaw PD con : slrealtimeloglib/File Log  decimation=1
      settings: SourceProductBaseCode=XP
  torque_x : Outport  PortDimensions=1  VectorParamsAs1DForOutWhenUnconnected=off
  torque_y : Outport  Port=2  PortDimensions=1  VectorParamsAs1DForOutWhenUnconnected=off
  torque_z : Outport  Port=3  PortDimensions=1  VectorParamsAs1DForOutWhenUnconnected=off
  F : Outport  Port=4  VectorParamsAs1DForOutWhenUnconnected=off
  att_e : Outport  Port=5  PortDimensions=3  VectorParamsAs1DForOutWhenUnconnected=off
  alt_e : Outport  Port=6  VectorParamsAs1DForOutWhenUnconnected=off
  wires:
  r/1 -> RTMPC Trajectory Tracking/2(r)
  r_dot/1 -> RTMPC Trajectory Tracking/3(r_dot)
  r_dotdot/1 -> RTMPC Trajectory Tracking/4(r_dotdot)
  R/1 -> Geometric Attitude Controller/2(R), Scope1/1, Rotm2rpy1/1(R), RTMPC Trajectory Tracking/5(R)
  Omega/1 -> Geometric Attitude Controller/3(Omega), RTMPC Trajectory Tracking/6(Omega), External Torque Observer/2(omega), Scope7/1
  rd/1 -> RTMPC Trajectory Tracking/7(rd)
  rd_d/1 -> RTMPC Trajectory Tracking/8(rd_d)
  rd_dd/1 -> RTMPC Trajectory Tracking/9(rd_dd)
  Geometric Attitude Controller/2(att_e) -> Scope3/1, To Workspace/1, att_e/1
  rd_ddd/1 -> RTMPC Trajectory Tracking/10(rd_ddd)
  rd_dddd/1 -> RTMPC Trajectory Tracking/11(rd_dddd)
  int_e/1 -> RTMPC Trajectory Tracking/13(int_e)
  RTMPC Trajectory Tracking/3(cmd_B_acc_z) -> Mux/2, To Workspace6/1, F/1
  RTMPC Trajectory Tracking/4(alt_e) -> alt_e/1
  time/1(real times) -> External Torque Observer/1(time), MATLAB Function/3(time), Geometric Attitude Controller/1(time), RTMPC Trajectory Tracking/1(time)
  RTMPC Trajectory Tracking/1(Rd) -> Scope2/1, Geometric Attitude Controller/4(Rd), Rotm2rpy/1(R)
  RTMPC Trajectory Tracking/2(Omegad) -> Geometric Attitude Controller/5(Omegad), Mux1/5, To Workspace4/1
  Rotm2rpy1/1(rpy) -> Mux1/3, To Workspace2/1
  RTMPC Trajectory Tracking/5(rd_rtmpc) -> Mux1/2, To Workspace3/1
  Demux/2 -> torque_y/1, MATLAB Function/2(Ty)
  Demux/3 -> torque_z/1
  Geometric Attitude Controller/1(cmd_B_torque) -> Demux/1, Mux1/4, To Workspace5/1, Scope/1
  Rotm2rpy/1(rpy) -> Mux/1
  External Torque Observer/1(omega_hat) -> Delay1/1
  External Torque Observer/2(ext_torque_hat) -> Mux1/6, Delay/1
  Delay/1 -> Saturation/1, External Torque Observer/5("ext_torque_hat "), Scope4/1
  Delay1/1 -> Scope5/1, External Torque Observer/6("omega_hat ")
  Demux/1 -> MATLAB Function/1(Tx), torque_x/1
  Multiply/1 -> Geometric Attitude Controller/6(tau_ext)
  RTMPC Trajectory Tracking/6(new_att_cmd) -> Delay2/1
  Delay2/1 -> RTMPC Trajectory Tracking/12(att_cmd)
  Mux/1 -> Mux1/1, To Workspace1/1
  Mux1/1 -> yaw PD con/1
  MATLAB Function/1(Tx_out) -> External Torque Observer/3(torque_x), Scope6/1
  MATLAB Function/2(Ty_out) -> Scope8/1, External Torque Observer/4(torque_y)
  Saturation/1 -> Mux1/7, Multiply/1

== system controller_v13/Adaptive Controller/adaptive system ==
  att_e : Inport
  alt_e : Inport  Port=2
  Mux : Mux  Inputs=2
  Saturation1 : Saturate  UpperLimit=1  LowerLimit=-1
  Saturation3 : Saturate  UpperLimit=0.06  LowerLimit=-0.06
  Scope : Scope
  Unit Delay : UnitDelay  SampleTime=-1  HasFrameUpgradeWarning=on
  enable1 : Product  Inputs=**
  integral enable : Constant  Value=ctr.integral.en
  integrator : Subsystem
  safety1 : Subsystem
  safety2 : Subsystem
  thrust offset : Constant  Value=flt.thrust_off
  torque offset : Constant  Value=[flt.torx_off;flt.tory_off;flt.torz_off]
  " tor_off" : Outport
  th_off : Outport  Port=2
  int_e : Outport  Port=3
  wires:
  torque offset/1 -> integrator/2(torque offset)
  thrust offset/1 -> integrator/3(thrust_offset)
  integrator/3(th_off) -> th_off/1
  integrator/1(int_e) -> Unit Delay/1
  integral enable/1 -> enable1/1
  Mux/1 -> integrator/1(e)
  Unit Delay/1 -> enable1/2
  integrator/2(" torq_off") -> Scope/1, " tor_off"/1
  att_e/1 -> safety1/1(In1)
  enable1/1 -> int_e/1
  alt_e/1 -> safety2/1(In1)
  Saturation1/1 -> Mux/1
  Saturation3/1 -> Mux/2
  safety1/1(Out1) -> Saturation1/1
  safety2/1(Out1) -> Saturation3/1

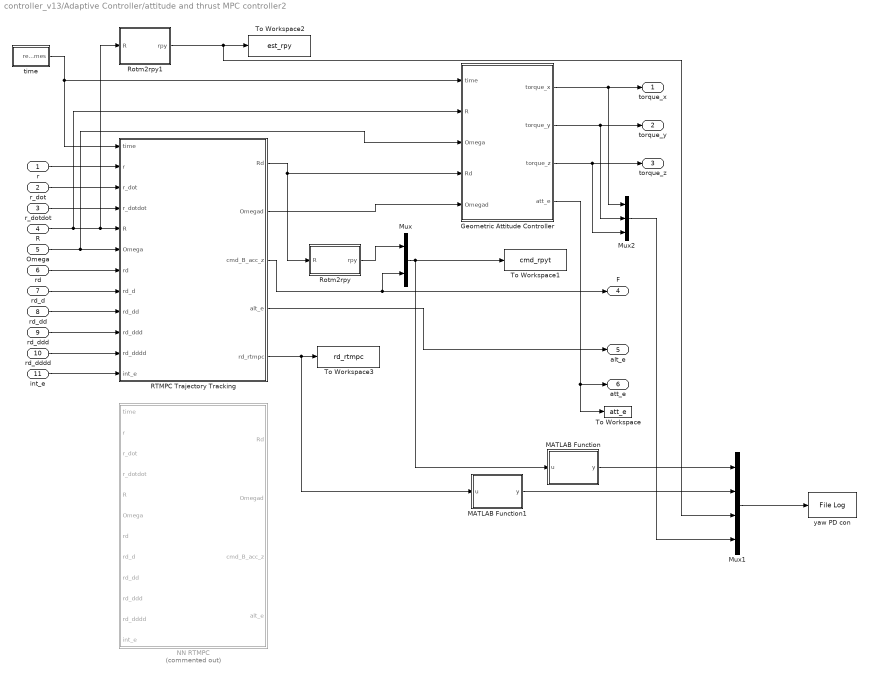
== system controller_v13/Adaptive Controller/attitude and thrust MPC controller2 ==
  r : Inport
  r_dot : Inport  Port=2
  r_dotdot : Inport  Port=3
  R : Inport  Port=4
  Omega : Inport  Port=5  PortDimensions=3
  rd : Inport  Port=6
  rd_d : Inport  Port=7
  rd_dd : Inport  Port=8
  rd_ddd : Inport  Port=9
  rd_dddd : Inport  Port=10
  int_e : Inport  Port=11
  Geometric Attitude Controller : MATLAB Function  TreatAsAtomicUnit=on  SystemSampleTime=mdl.T
  MATLAB Function : MATLAB Function  TreatAsAtomicUnit=on  SystemSampleTime=mdl.T
  MATLAB Function1 : MATLAB Function  TreatAsAtomicUnit=on  SystemSampleTime=mdl.T
  Mux : Mux  Inputs=2
  Mux1 : Mux
  Mux2 : Mux  Inputs=3
  NN RTMPC : Subsystem  Commented=on
  RTMPC Trajectory Tracking : MATLAB Function  TreatAsAtomicUnit=on  SystemSampleTime=0.01
  Rotm2rpy : MATLAB Function  TreatAsAtomicUnit=on  SystemSampleTime=0.01
  Rotm2rpy1 : MATLAB Function  TreatAsAtomicUnit=on
  To Workspace : ToWorkspace  VariableName=att_e  SaveFormat=Timeseries  SampleTime=-1
  To Workspace1 : ToWorkspace  VariableName=cmd_rpyt  SaveFormat=Timeseries  SampleTime=-1
  To Workspace2 : ToWorkspace  VariableName=est_rpy  SaveFormat=Timeseries  SampleTime=-1
  To Workspace3 : ToWorkspace  VariableName=rd_rtmpc  SaveFormat=Timeseries  SampleTime=-1
  time : Subsystem
  yaw PD con : slrealtimeloglib/File Log  decimation=1
      settings: SourceProductBaseCode=XP
  torque_x : Outport  PortDimensions=1  VectorParamsAs1DForOutWhenUnconnected=off
  torque_y : Outport  Port=2  PortDimensions=1  VectorParamsAs1DForOutWhenUnconnected=off
  torque_z : Outport  Port=3  PortDimensions=1  VectorParamsAs1DForOutWhenUnconnected=off
  F : Outport  Port=4  VectorParamsAs1DForOutWhenUnconnected=off
  alt_e : Outport  Port=5  VectorParamsAs1DForOutWhenUnconnected=off
  att_e : Outport  Port=6  PortDimensions=3  VectorParamsAs1DForOutWhenUnconnected=off
  wires:
  r/1 -> RTMPC Trajectory Tracking/2(r)
  r_dot/1 -> RTMPC Trajectory Tracking/3(r_dot)
  r_dotdot/1 -> RTMPC Trajectory Tracking/4(r_dotdot)
  R/1 -> Geometric Attitude Controller/2(R), RTMPC Trajectory Tracking/5(R), Rotm2rpy1/1(R)
  Omega/1 -> RTMPC Trajectory Tracking/6(Omega), Geometric Attitude Controller/3(Omega)
  rd/1 -> RTMPC Trajectory Tracking/7(rd)
  rd_d/1 -> RTMPC Trajectory Tracking/8(rd_d)
  rd_dd/1 -> RTMPC Trajectory Tracking/9(rd_dd)
  Geometric Attitude Controller/4(att_e) -> att_e/1, To Workspace/1
  rd_ddd/1 -> RTMPC Trajectory Tracking/10(rd_ddd)
  rd_dddd/1 -> RTMPC Trajectory Tracking/11(rd_dddd)
  int_e/1 -> RTMPC Trajectory Tracking/12(int_e)
  Geometric Attitude Controller/1(torque_x) -> Mux2/1, torque_x/1
  Geometric Attitude Controller/2(torque_y) -> Mux2/2, torque_y/1
  Geometric Attitude Controller/3(torque_z) -> Mux2/3, torque_z/1
  RTMPC Trajectory Tracking/3(cmd_B_acc_z) -> Mux/2, F/1
  Mux/1 -> To Workspace1/1, MATLAB Function/1(u)
  RTMPC Trajectory Tracking/4(alt_e) -> alt_e/1
  time/1(real times) -> RTMPC Trajectory Tracking/1(time), Geometric Attitude Controller/1(time)
  RTMPC Trajectory Tracking/1(Rd) -> Rotm2rpy/1(R), Geometric Attitude Controller/4(Rd)
  RTMPC Trajectory Tracking/2(Omegad) -> Geometric Attitude Controller/5(Omegad)
  Rotm2rpy/1(rpy) -> Mux/1
  Rotm2rpy1/1(rpy) -> Mux1/3, To Workspace2/1
  RTMPC Trajectory Tracking/5(rd_rtmpc) -> MATLAB Function1/1(u), To Workspace3/1
  Mux1/1 -> yaw PD con/1
  Mux2/1 -> Mux1/4
  MATLAB Function/1(y) -> Mux1/1
  MATLAB Function1/1(y) -> Mux1/2

== system controller_v13/Adaptive Controller/attitude and thrust controller1 ==
  r : Inport
  r_dot : Inport  Port=2
  r_dotdot : Inport  Port=3
  R : Inport  Port=4
  Omega : Inport  Port=5
  rd : Inport  Port=6
  rd_d : Inport  Port=7
  rd_dd : Inport  Port=8
  rd_ddd : Inport  Port=9
  rd_dddd : Inport  Port=10
  int_e : Inport  Port=11
  Attitude Controleller : MATLAB Function  TreatAsAtomicUnit=on
  Constant : Constant
  Thrust Controller : MATLAB Function  TreatAsAtomicUnit=on
  yaw PD con : slrealtimeloglib/File Log  decimation=1
      settings: SourceProductBaseCode=XP
  torque_x : Outport
  torque_y : Outport  Port=2
  torque_z : Outport  Port=3
  F : Outport  Port=4
  att_e : Outport  Port=5
  alt_e : Outport  Port=6
  wires:
  r/1 -> Thrust Controller/1(r), Attitude Controleller/1(r)
  Attitude Controleller/1(torque_x) -> torque_x/1
  r_dot/1 -> Attitude Controleller/2(r_dot), Thrust Controller/2(r_dot)
  r_dotdot/1 -> Attitude Controleller/3(r_dotdot), Thrust Controller/3(r_dotdot)
  R/1 -> Attitude Controleller/4(R), Thrust Controller/4(R)
  Attitude Controleller/2(torque_y) -> torque_y/1
  Omega/1 -> Attitude Controleller/5(Omega), Thrust Controller/5(Omega)
  rd/1 -> Attitude Controleller/6(rd), Thrust Controller/6(rd)
  rd_d/1 -> Attitude Controleller/7(rd_d), Thrust Controller/7(rd_d)
  rd_dd/1 -> Attitude Controleller/8(rd_dd), Thrust Controller/8(rd_dd)
  Attitude Controleller/4(att_e) -> att_e/1
  rd_ddd/1 -> Attitude Controleller/9(rd_ddd), Thrust Controller/9(rd_ddd)
  rd_dddd/1 -> Attitude Controleller/10(rd_dddd), Thrust Controller/10(rd_dddd)
  int_e/1 -> Attitude Controleller/11(int_e), Thrust Controller/11(int_e)
  Thrust Controller/2(alt_e) -> alt_e/1
  Thrust Controller/1(F) -> F/1
  Attitude Controleller/3(torque_z) -> torque_z/1
  Constant/1 -> yaw PD con/1
